simulink model "（旧）PCM_Noisy"  (R2018a)
settings: Solver=ode45  StartTime=0.0  StopTime=1  RelTol=1e-3  EnableMultiTasking=on
undefined symbols (not defined in the file): bchgenpoly
libraries: commdigbbndpm3 x2, commblkcod2 x2, commsrccod2 x2, commutil2 x2, commsink2 x1, commchan3 x1, dsparch4 x1, dspobslib x1
settings Model: Creator=www  LastModifiedBy=ddd
settings DataIOCC: LimitDataPoints=on  SaveFormat=Array
settings OptimizationCC: LifeSpan=inf
settings DebuggingCC: SolverPrmCheckMsg=warning  SFUnexpectedBacktrackingDiag=warning  SFNoUnconditionalDefaultTransitionDiag=warning  SFExecutionAtInitializationDiag=none
settings HardwareCC: ProdBitPerPointer=32  ProdBitPerSizeT=32  ProdBitPerPtrDiffT=32  ProdLargestAtomicFloat=None  ProdIntDivRoundTo=Undefined  ProdEndianess=Unspecified  ProdWordSize=32  ProdHWDeviceType=32-bit Generic
settings ModelReferenceCC: PropagateSignalLabelsOutOfModel=off
settings CodeAppCC: StateflowObjectComments=on
settings GRTTargetCC: TargetLangStandard=C89/C90 (ANSI)  GeneratePreprocessorConditionals=Disable all
settings ConfigComp: CovMetricSettings=dw  CovHtmlReporting=on  CovSaveCumulativeToWorkspaceVar=on  CovSaveSingleToWorkspaceVar=on  CovExternalEMLEnable=off  CovSFcnEnable=off

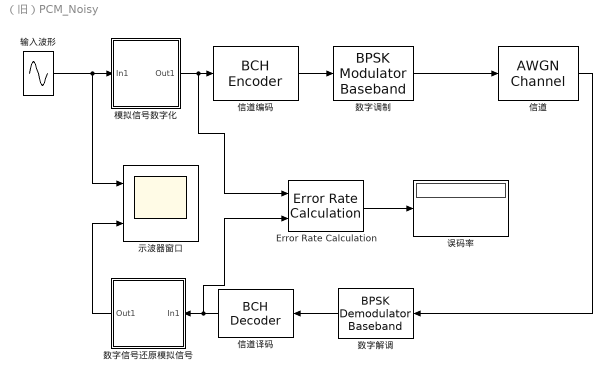
== system （旧）PCM_Noisy ==
  " 数字调制" : commdigbbndpm3/BPSK Modulator Baseband  Ph=0  outDtype=double  outWordLen=16  outUDDataType=sfix(16)  outFracLenMode=Best precision  outFracLen=15  outDataTypeStr=double  outLastDataTypeStr=double
  Error Rate Calculation : commsink2/Error Rate Calculation  N=0  st_delay=0  cp_mode=Entire frame  subframe=[]  PMode=Port  WsName=ErrorVec  RsMode2=off  stop=off  numErr=100  maxBits=1e6
  信道 : commchan3/AWGN Channel  InputProcessing=Columns as channels (frame based)  seed=67  noiseMode="Signal to noise ratio  (SNR)"  EbNodB=30  EsNodB=20  SNRdB=1  bitsPerSym=1  Ps=1  Tsym=1  variance=1
  信道编码 : commblkcod2/BCH Encoder  n=4  k=1  specShortening=off  shortenedK=5  specGenPoly=off  genPoly=bchgenpoly(15,5)  specPrimPoly=off  prPoly=[1 0 0 1 1]  specDisableGenCheck=off  specPuncture=off  punctVec=[ones(8,1); zeros(2,1)]
      settings: SourceProductName=Communications System Toolbox  SourceProductBaseCode=CM
  信道译码 : commblkcod2/BCH Decoder  n=4  k=1  specShortening=off  shortenedK=5  specGenPoly=off  genPoly=bchgenpoly(15,5)  specPrimPoly=off  prPoly=[1 0 0 1 1]  specDisableGenCheck=off  specPuncture=off  punctVec=[ones(8,1); zeros(2,1)]  specErasurePort=off  showNumErr=off
      settings: SourceProductName=Communications System Toolbox  SourceProductBaseCode=CM
  数字信号还原模拟信号 : Subsystem
  数字解调 : commdigbbndpm3/BPSK Demodulator Baseband  DecType=Hard decision  VarSource=Dialog  Variance=1  Ph=0  outDtype=Inherit via internal rule  derotateFactorWordLen=16  derotateFactorDataTypeStr=Inherit: Same word length as input  derotateFactorLastDataTypeStr=Inherit: Same word length as input
  模拟信号数字化 : Subsystem
  示波器窗口 : Scope  NumInputPorts=2
  误码率 : Display
  输入波形 : Sin  Frequency=100*2*pi  SampleTime=0
  wires:
  输入波形/1 -> 示波器窗口/1, 模拟信号数字化/1(In1)
  " 数字调制"/1 -> 信道/1
  信道/1 -> 数字解调/1
  模拟信号数字化/1(Out1) -> Error Rate Calculation/1, 信道编码/1
  信道编码/1 -> " 数字调制"/1
  数字解调/1 -> 信道译码/1
  信道译码/1 -> Error Rate Calculation/2, 数字信号还原模拟信号/1(In1)
  数字信号还原模拟信号/1(Out1) -> 示波器窗口/2
  Error Rate Calculation/1 -> 误码率/1

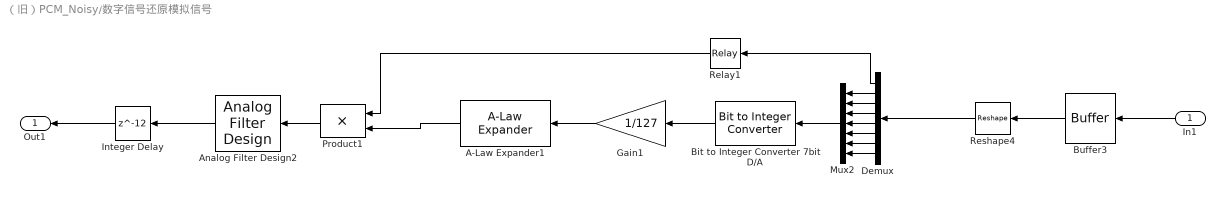
== system （旧）PCM_Noisy/数字信号还原模拟信号 ==
  In1 : Inport
  A-Law Expander1 : commsrccod2/A-Law Expander  A=87.6  V=1
      settings: SourceProductName=Communications System Toolbox  SourceProductBaseCode=CM
  Analog Filter Design2 : dsparch4/Analog Filter Design  method=Butterworth  filttype=Lowpass  N=8  Wlo=250*pi  Whi=80  Rp=2  Rs=40
  Bit to Integer Converter 7bit D/A : commutil2/Bit to Integer Converter  nbits=7  bitOrder=MSB first  signedOutputValues=Unsigned  outDtype=Inherit via internal rule  outDtypeSigned=Inherit via internal rule
  Buffer3 : Buffer  N=8
  Demux : Demux  Outputs=8
  Gain1 : Gain  Gain=1/127  SaturateOnIntegerOverflow=on  OutDataTypeStr=Inherit: Same as input  ParamDataTypeStr=Inherit: Same as input
  Integer Delay : Delay  DelayLength=12  InputProcessing=Inherited  SampleTime=0.0001
  Mux2 : Mux  Inputs=7
  Product1 : Product  SaturateOnIntegerOverflow=on  OutDataTypeStr=Inherit: Same as first input
  Relay1 : Relay  OffOutputValue=-1
  Reshape4 : Reshape  OutputDimensions=[8,1]
  Out1 : Outport
  wires:
  Reshape4/1 -> Demux/1
  Product1/1 -> Analog Filter Design2/1
  Demux/4 -> Mux2/3
  A-Law Expander1/1 -> Product1/2
  Demux/5 -> Mux2/4
  Bit to Integer Converter 7bit D/A/1 -> Gain1/1
  Buffer3/1 -> Reshape4/1
  Relay1/1 -> Product1/1
  Integer Delay/1 -> Out1/1
  Gain1/1 -> A-Law Expander1/1
  Mux2/1 -> Bit to Integer Converter 7bit D/A/1
  Demux/2 -> Mux2/1
  In1/1 -> Buffer3/1
  Demux/1 -> Relay1/1
  Analog Filter Design2/1 -> Integer Delay/1
  Demux/6 -> Mux2/5
  Demux/7 -> Mux2/6
  Demux/3 -> Mux2/2
  Demux/8 -> Mux2/7

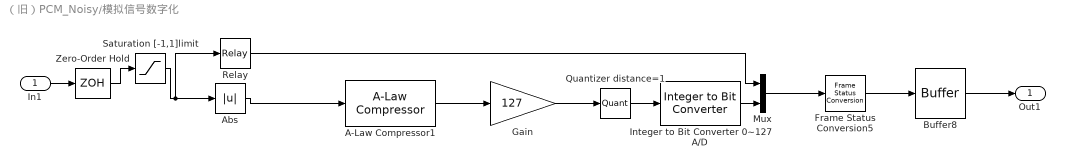
== system （旧）PCM_Noisy/模拟信号数字化 ==
  In1 : Inport
  A-Law Compressor1 : commsrccod2/A-Law Compressor  A=87.6  V=1
      settings: SourceProductName=Communications System Toolbox  SourceProductBaseCode=CM
  Abs : Abs  SaturateOnIntegerOverflow=on
  Buffer8 : Buffer  N=1
  Frame Status Conversion5 : dspobslib/Frame Status Conversion  growRefPort=off  outframe=Frame-based
      settings: SourceProductName=DSP System Toolbox  SourceProductBaseCode=DS
  Gain : Gain  Gain=127  SaturateOnIntegerOverflow=on  OutDataTypeStr=Inherit: Same as input  ParamDataTypeStr=Inherit: Same as input
  Integer to Bit Converter 0~127 A/D : commutil2/Integer to Bit Converter  nbits=7  signedInputValues=Unsigned  bitOrder=MSB first  outDtype=Inherit via internal rule
  Mux : Mux  Inputs=2
  Quantizer distance=1 : Quantizer  QuantizationInterval=1
  Relay : Relay
  Saturation [-1,1]limit : Saturate  UpperLimit=1  LowerLimit=-1
  Zero-Order Hold : ZeroOrderHold  SampleTime=0.001
  Out1 : Outport
  wires:
  Integer to Bit Converter 0~127 A/D/1 -> Mux/2
  Quantizer distance=1/1 -> Integer to Bit Converter 0~127 A/D/1
  Abs/1 -> A-Law Compressor1/1
  Frame Status Conversion5/1 -> Buffer8/1
  Zero-Order Hold/1 -> Saturation [-1,1]limit/1
  In1/1 -> Zero-Order Hold/1
  Mux/1 -> Frame Status Conversion5/1
  A-Law Compressor1/1 -> Gain/1
  Gain/1 -> Quantizer distance=1/1
  Saturation [-1,1]limit/1 -> Abs/1, Relay/1
  Relay/1 -> Mux/1
  Buffer8/1 -> Out1/1
